simulink model "TD_2doF"  (R2019b)
settings: Solver=VariableStepAuto  StartTime=0.0  StopTime=50  RelTol=1e-3
undefined symbols (not defined in the file): Dm, Dt, g, J_eq, K_pitch, Mb, w0_neg, w0_pos, w1_neg, w1_pos, w2_neg, w2_pos
settings Model: Creator=peter  LastModifiedBy=lbend

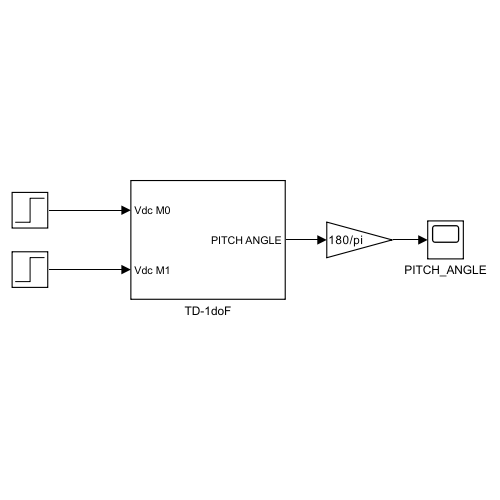
[thumbnail: Simulink's stored preview of the top-level diagram]
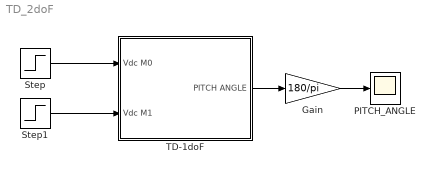
== system TD_2doF ==
  Gain : Gain  Gain=180/pi
  PITCH_ANGLE : Scope
  Step : Step  SampleTime=0
  Step1 : Step  SampleTime=0
  TD-1doF : Subsystem
  wires:
  TD-1doF/1(PITCH ANGLE) -> Gain/1
  Gain/1 -> PITCH_ANGLE/1
  Step1/1 -> TD-1doF/2(Vdc M1)
  Step/1 -> TD-1doF/1(Vdc M0)

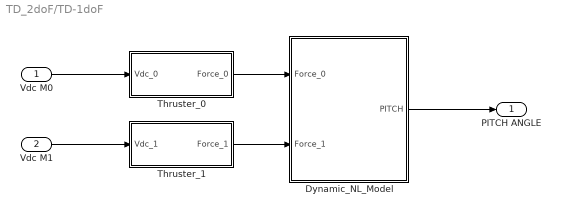
== system TD_2doF/TD-1doF ==
  Vdc M0 : Inport
  Vdc M1 : Inport  Port=2
  Dynamic_NL_Model : Subsystem
  Thruster_0 : Subsystem
  Thruster_1 : Subsystem
  PITCH ANGLE : Outport
  wires:
  Vdc M0/1 -> Thruster_0/1(Vdc_0)
  Dynamic_NL_Model/1(PITCH) -> PITCH ANGLE/1
  Thruster_1/1(Force_1) -> Dynamic_NL_Model/2("Force_1 ")
  Vdc M1/1 -> Thruster_1/1(Vdc_1)
  Thruster_0/1(Force_0) -> Dynamic_NL_Model/1(Force_0)

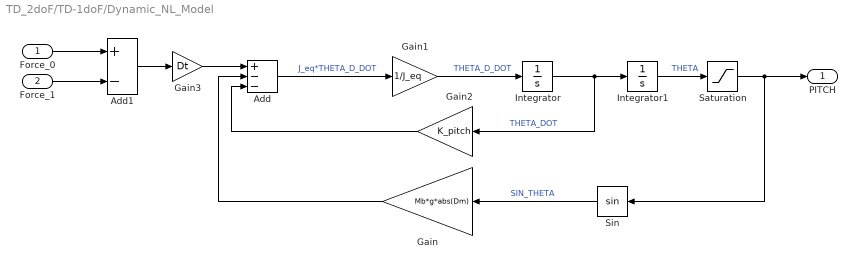
== system TD_2doF/TD-1doF/Dynamic_NL_Model ==
  Force_0 : Inport
  "Force_1 " : Inport  Port=2
  Add : Sum  Inputs=+--
  Add1 : Sum  Inputs=+-
  Gain : Gain  Gain=Mb*g*abs(Dm)
  Gain1 : Gain  Gain=1/J_eq
  Gain2 : Gain  Gain=K_pitch
  Gain3 : Gain  Gain=Dt
  Integrator : Integrator
  Integrator1 : Integrator
  Saturation : Saturate  UpperLimit=0.93  LowerLimit=-0.93
  Sin : Trigonometry
  PITCH : Outport
  wires:
  Gain3/1 -> Add/1
  Gain2/1 -> Add/3
  Add/1 -> Gain1/1  "J_eq*THETA_D_DOT"
  Integrator1/1 -> Saturation/1  "THETA"
  "Force_1 "/1 -> Add1/2
  Gain/1 -> Add/2
  Add1/1 -> Gain3/1
  Force_0/1 -> Add1/1
  Gain1/1 -> Integrator/1  "THETA_D_DOT"
  Sin/1 -> Gain/1  "SIN_THETA"
  Integrator/1 -> Gain2/1, Integrator1/1  "THETA_DOT"
  Saturation/1 -> Sin/1, PITCH/1

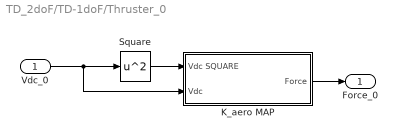
== system TD_2doF/TD-1doF/Thruster_0 ==
  Vdc_0 : Inport
  K_aero MAP : Subsystem
  Square : Math  Operator=square  SaturateOnIntegerOverflow=on
  Force_0 : Outport
  wires:
  Vdc_0/1 -> K_aero MAP/2(Vdc), Square/1
  Square/1 -> K_aero MAP/1(Vdc SQUARE)
  K_aero MAP/1(Force) -> Force_0/1

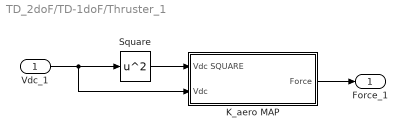
== system TD_2doF/TD-1doF/Thruster_1 ==
  Vdc_1 : Inport
  K_aero MAP : Subsystem
  Square : Math  Operator=square  SaturateOnIntegerOverflow=on
  Force_1 : Outport
  wires:
  Vdc_1/1 -> K_aero MAP/2(Vdc), Square/1
  Square/1 -> K_aero MAP/1(Vdc SQUARE)
  K_aero MAP/1(Force) -> Force_1/1

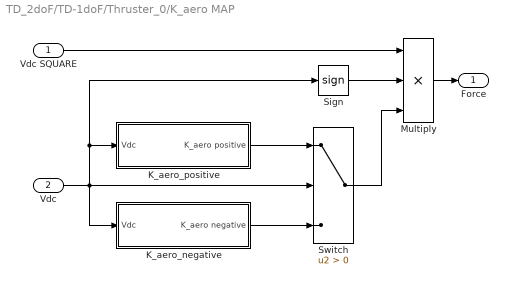
== system TD_2doF/TD-1doF/Thruster_0/K_aero MAP ==
  Vdc SQUARE : Inport
  Vdc : Inport  Port=2
  K_aero_negative : Subsystem
  K_aero_positive : Subsystem
  "Multiply " : Product  Inputs=***
  Sign : Signum
  Switch : Switch  Criteria=u2 > Threshold
  Force : Outport
  wires:
  Vdc SQUARE/1 -> "Multiply "/1
  "Multiply "/1 -> Force/1
  Vdc/1 -> K_aero_negative/1(Vdc), Switch/2, Sign/1, K_aero_positive/1(Vdc)
  K_aero_positive/1(K_aero positive) -> Switch/1
  K_aero_negative/1(K_aero negative) -> Switch/3
  Switch/1 -> "Multiply "/3
  Sign/1 -> "Multiply "/2

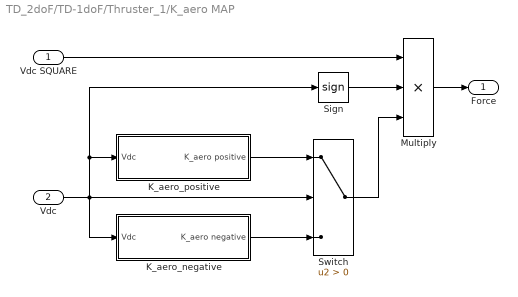
== system TD_2doF/TD-1doF/Thruster_1/K_aero MAP ==
  Vdc SQUARE : Inport
  Vdc : Inport  Port=2
  K_aero_negative : Subsystem
  K_aero_positive : Subsystem
  "Multiply " : Product  Inputs=***
  Sign : Signum
  Switch : Switch  Criteria=u2 > Threshold
  Force : Outport
  wires:
  Vdc SQUARE/1 -> "Multiply "/1
  "Multiply "/1 -> Force/1
  K_aero_positive/1(K_aero positive) -> Switch/1
  K_aero_negative/1(K_aero negative) -> Switch/3
  Switch/1 -> "Multiply "/3
  Sign/1 -> "Multiply "/2
  Vdc/1 -> K_aero_negative/1(Vdc), Switch/2, Sign/1, K_aero_positive/1(Vdc)

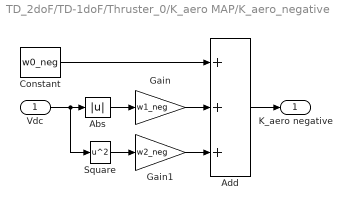
== system TD_2doF/TD-1doF/Thruster_0/K_aero MAP/K_aero_negative ==
  Vdc : Inport
  Abs : Abs
  Add : Sum  Inputs=+++
  Constant : Constant  Value=w0_neg
  Gain : Gain  Gain=w1_neg
  Gain1 : Gain  Gain=w2_neg
  Square : Math  Operator=square  SaturateOnIntegerOverflow=on
  K_aero negative : Outport
  wires:
  Gain1/1 -> Add/3
  Add/1 -> K_aero negative/1
  Constant/1 -> Add/1
  Gain/1 -> Add/2
  Square/1 -> Gain1/1
  Abs/1 -> Gain/1
  Vdc/1 -> Square/1, Abs/1

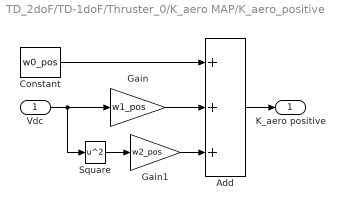
== system TD_2doF/TD-1doF/Thruster_0/K_aero MAP/K_aero_positive ==
  Vdc : Inport
  Add : Sum  Inputs=+++
  Constant : Constant  Value=w0_pos
  Gain : Gain  Gain=w1_pos
  Gain1 : Gain  Gain=w2_pos
  Square : Math  Operator=square  SaturateOnIntegerOverflow=on
  K_aero positive : Outport
  wires:
  Constant/1 -> Add/1
  Vdc/1 -> Square/1, Gain/1
  Add/1 -> K_aero positive/1
  Gain/1 -> Add/2
  Square/1 -> Gain1/1
  Gain1/1 -> Add/3

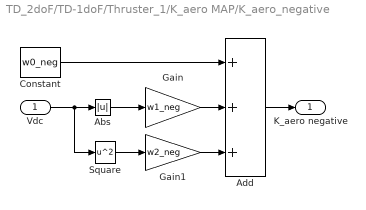
== system TD_2doF/TD-1doF/Thruster_1/K_aero MAP/K_aero_negative ==
  Vdc : Inport
  Abs : Abs
  Add : Sum  Inputs=+++
  Constant : Constant  Value=w0_neg
  Gain : Gain  Gain=w1_neg
  Gain1 : Gain  Gain=w2_neg
  Square : Math  Operator=square  SaturateOnIntegerOverflow=on
  K_aero negative : Outport
  wires:
  Gain1/1 -> Add/3
  Add/1 -> K_aero negative/1
  Constant/1 -> Add/1
  Gain/1 -> Add/2
  Square/1 -> Gain1/1
  Abs/1 -> Gain/1
  Vdc/1 -> Square/1, Abs/1

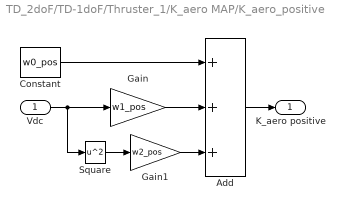
== system TD_2doF/TD-1doF/Thruster_1/K_aero MAP/K_aero_positive ==
  Vdc : Inport
  Add : Sum  Inputs=+++
  Constant : Constant  Value=w0_pos
  Gain : Gain  Gain=w1_pos
  Gain1 : Gain  Gain=w2_pos
  Square : Math  Operator=square  SaturateOnIntegerOverflow=on
  K_aero positive : Outport
  wires:
  Constant/1 -> Add/1
  Vdc/1 -> Square/1, Gain/1
  Add/1 -> K_aero positive/1
  Gain/1 -> Add/2
  Square/1 -> Gain1/1
  Gain1/1 -> Add/3
